simulink model "gouskov"  (Simulink 10.2)
settings: Solver=ode45  StartTime=0.0  StopTime=100.0  MaxStep=0.01  RelTol=1e-3  EnableMultiTasking=on
values from neighbouring files (symbols this model uses):
  a11 = 0.642    [Lab_rab_3.m]
  a21 = 5.65    [Lab_rab_3.m]
  a22 = 0.468    [Lab_rab_3.m]
  a46 = 168    [Lab_rab_3.m]
  a51 = 11    [Lab_rab_3.m]
  b2 = 4.9    [Lab_rab_3.m]
  DHz = 100    [Lab_rab_3.m]
  f = 0    [Lab_rab_3.m]
  Ih = 0    [Lab_rab_3.m]
  Ip = 0. ���������� f = 0\n')    [Lab_rab_3.m]
  Ktet = input('������� �������� ������������ Ktet: ')    [Lab_rab_3.m]
  Kwz = 0.4    [Lab_rab_3.m]
  N_of_var = input('Задай вариант, пёс: ')    [Lab_rab_3.m]
settings Model: Creator=Администратор  LastModifiedBy=Администратор  ExtModeTrigMode=oneshot  ExtModeArmWhenConnect=off
settings OptimizationCC: BlockReduction=off  BooleanDataType=off  LifeSpan=auto
settings DebuggingCC: SaveWithParameterizedLinksMsg=none  SignalResolutionControl=TryResolveAllWithWarning  MultiTaskDSMMsg=warning  MultiTaskCondExecSysMsg=none  FcnCallInpInsideContextMsg=error  SFUnexpectedBacktrackingDiag=error  SFNoUnconditionalDefaultTransitionDiag=error  SFExecutionAtInitializationDiag=warning  ArithmeticOperatorsInVariantConditions=error
settings HardwareCC: ProdBitPerPointer=64  ProdBitPerSizeT=64  ProdBitPerPtrDiffT=64  ProdLargestAtomicFloat=Float  ProdIntDivRoundTo=Zero  ProdEndianess=LittleEndian  ProdWordSize=64  ProdHWDeviceType=Intel->x86-64 (Windows64)  TargetUnknown=on
settings SFSimCC: SimUseLocalCustomCode=on  CustomCodeUndefinedFunction=FilterOut
settings RTWCC: RTWUseLocalCustomCode=on
settings CodeAppCC: StateflowObjectComments=off
settings GRTTargetCC: TargetLangStandard=C99 (ISO)
settings ConfigComp: CovMetricSettings=dwe  CovSaveCumulativeToWorkspaceVar=off  CovSaveSingleToWorkspaceVar=off  CovExternalEMLEnable=on

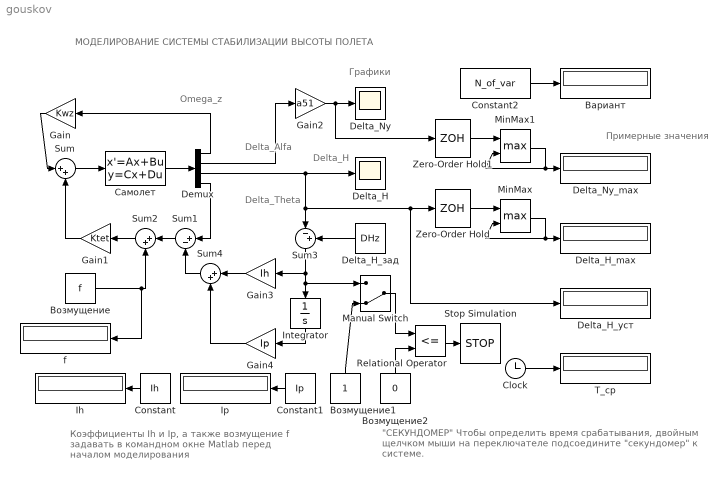
== system gouskov ==
  note: МОДЕЛИРОВАНИЕ СИСТЕМЫ СТАБИЛИЗАЦИИ ВЫСОТЫ ПОЛЕТА
  note: Примерные
      | значения
  note: Графики
  note: Omega_z
  note: Delta_H
  note: Delta_Alfa
  note: Delta_Theta
  note: Коэффициенты Ih и Ip, а также возмущение f
      | задавать в командном окне Matlab
      | перед началом моделирования
  note: "СЕКУНДОМЕР"
      | Чтобы определить время срабатывания, двойным щелчком мыши
      | на переключателе подсоедините "секундомер" к системе.
  Clock : Clock
  Constant : Constant  Value=Ih
  Constant1 : Constant  Value=Ip
  Constant2 : Constant  Value=N_of_var
  Delta_H : Scope
  Delta_H_max : Display
  Delta_H_зад : Constant  Value=DHz
  Delta_H_уст : Display
  Delta_Ny : Scope
  Delta_Ny_max : Display
  Demux : Demux
  Gain : Gain  Gain=Kwz  SaturateOnIntegerOverflow=on
  Gain1 : Gain  Gain=Ktet  SaturateOnIntegerOverflow=on
  Gain2 : Gain  Gain=a51  SaturateOnIntegerOverflow=on
  Gain3 : Gain  Gain=Ih  SaturateOnIntegerOverflow=on
  Gain4 : Gain  Gain=Ip  SaturateOnIntegerOverflow=on
  Ih : Display
  Integrator : Integrator
  Ip : Display
  Manual Switch : ManualSwitch  CurrentSetting=0
  MinMax : MinMax  Function=max  Inputs=2
  MinMax1 : MinMax  Function=max  Inputs=2
  Relational Operator : RelationalOperator  Operator=<=  RndMeth=Nearest  InputSameDT=on
  Stop Simulation : Stop
  Sum : Sum  Inputs=|++  SaturateOnIntegerOverflow=on
  Sum1 : Sum  Inputs=|+-  SaturateOnIntegerOverflow=on
  Sum2 : Sum  Inputs=|++  SaturateOnIntegerOverflow=on
  Sum3 : Sum  Inputs=|-+  SaturateOnIntegerOverflow=on
  Sum4 : Sum  Inputs=|++  SaturateOnIntegerOverflow=on
  T_cp : Display
  Zero-Order Hold : ZeroOrderHold
  Zero-Order Hold1 : ZeroOrderHold
  f : Display
  Вариант : Display
  Возмущение : Constant  Value=f
  Возмущение1 : Constant
  Возмущение2 : Constant  Value=0
  Самолет : StateSpace  A=[-a11 1 0 0; -a21 -a22 0 0; 0 1 0 0; -a46 1 a46 0]  B=[0; -b2; 0; 0]  C=[0 1 0 0; 1 0 0 0; 0 0 0 1;0 0 1 0]  D=[0; 0; 0; 0]  InitialCondition=0
  wires:
  Gain/1 -> Sum/1
  Gain1/1 -> Sum/2
  Sum/1 -> Самолет/1
  Самолет/1 -> Demux/1
  Sum1/1 -> Sum2/1
  Sum2/1 -> Gain1/1
  Integrator/1 -> Gain4/1
  Demux/1 -> Gain/1
  Demux/3 -> Delta_H/1, Sum3/1, Zero-Order Hold/1, Delta_H_уст/1
  Demux/4 -> Sum1/1
  Demux/2 -> Gain2/1
  Zero-Order Hold/1 -> MinMax/1
  MinMax/1 -> Delta_H_max/1, MinMax/2
  Zero-Order Hold1/1 -> MinMax1/1
  MinMax1/1 -> Delta_Ny_max/1, MinMax1/2
  Gain3/1 -> Sum4/1
  Sum4/1 -> Sum1/2
  Gain2/1 -> Zero-Order Hold1/1, Delta_Ny/1
  Delta_H_зад/1 -> Sum3/2
  Sum3/1 -> Gain3/1, Integrator/1, Manual Switch/1
  Manual Switch/1 -> Relational Operator/1
  Возмущение1/1 -> Manual Switch/2
  Возмущение2/1 -> Relational Operator/2
  Relational Operator/1 -> Stop Simulation/1
  Clock/1 -> T_cp/1
  Constant/1 -> Ih/1
  Gain4/1 -> Sum4/2
  Constant1/1 -> Ip/1
  Constant2/1 -> Вариант/1
  Возмущение/1 -> Sum2/2, f/1
